simulink model "differenzier_1"  (Simulink 5.0)
settings: Solver=ode45  StartTime=0.0  StopTime=10.0  RelTol=1e-3
undefined symbols (not defined in the file or in its folder): remez
libraries: dsparch4 x3, dspsigops x2
settings Model: Creator=svenhoffmann  LastModifiedBy=svenhoffmann  ExtModeAutoUpdateStatusClock=off

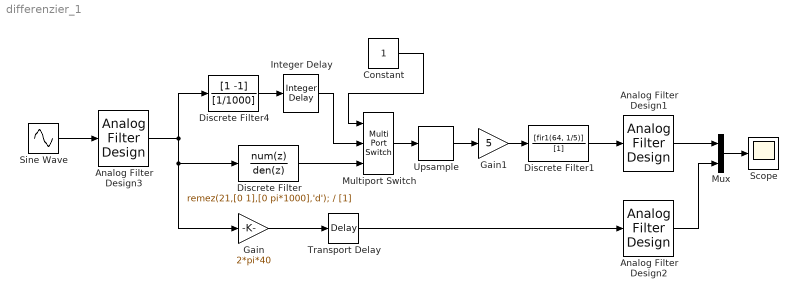
== system differenzier_1 ==
  Analog Filter Design1 : dsparch4/Analog Filter Design  method=Butterworth  filttype=Lowpass  N=8  Wlo=2*pi*1000  Whi=80  Rp=2  Rs=40
  Analog Filter Design2 : dsparch4/Analog Filter Design  method=Butterworth  filttype=Lowpass  N=8  Wlo=2*pi*1000  Whi=80  Rp=2  Rs=40
  Analog Filter Design3 : dsparch4/Analog Filter Design  method=Butterworth  filttype=Lowpass  N=8  Wlo=2*pi*450  Whi=80  Rp=2  Rs=40
  Constant : Constant
  Discrete Filter : DiscreteFilter  Numerator=remez(21,[0 1],[0 pi*1000],'d');  Denominator=[1]  SampleTime=1/1000
  Discrete Filter1 : DiscreteFilter  Numerator=[fir1(64, 1/5)]  Denominator=[1]  SampleTime=1/(5*1000)
  Discrete Filter4 : DiscreteFilter  Numerator=[1 -1]  Denominator=[1/1000]  SampleTime=1/1000
  Gain : Gain  Gain=2*pi*40  SaturateOnIntegerOverflow=on
  Gain1 : Gain  Gain=5  SaturateOnIntegerOverflow=on
  Integer Delay : dspsigops/Integer Delay  delay=11  ic=0  reset_popup=None
  Multiport Switch : MultiPortSwitch  Inputs=2  SaturateOnIntegerOverflow=on
  Mux : Mux  Inputs=2
  Scope : Scope
      settings: YMin=-275  YMax=300
  Sine Wave : Sin  Frequency=2*pi*40  SampleTime=0
  Transport Delay : TransportDelay  DelayTime=32.95/1000
  Upsample : dspsigops/Upsample  N=5  phase=0  ic=0  mode=Maintain input frame size
  wires:
  Sine Wave/1 -> Analog Filter Design3/1
  Mux/1 -> Scope/1
  Multiport Switch/1 -> Upsample/1
  Constant/1 -> Multiport Switch/1
  Discrete Filter4/1 -> Integer Delay/1
  Gain/1 -> Transport Delay/1
  Transport Delay/1 -> Analog Filter Design2/1
  Discrete Filter/1 -> Multiport Switch/3
  Integer Delay/1 -> Multiport Switch/2
  Analog Filter Design3/1 -> Discrete Filter4/1, Discrete Filter/1, Gain/1
  Analog Filter Design2/1 -> Mux/2
  Upsample/1 -> Gain1/1
  Gain1/1 -> Discrete Filter1/1
  Discrete Filter1/1 -> Analog Filter Design1/1
  Analog Filter Design1/1 -> Mux/1
